simulink model "version 1.0"  (R2020a)
settings: Solver=FixedStepAuto  StartTime=0.0  StopTime=10.0  FixedStep=1e-3  RelTol=1e-3  EnableMultiTasking=on
settings Model: ExtModeTrigDuration=5  Creator=qasim  LastModifiedBy=qasim
settings OptimizationCC: EnhancedBackFolding=on  PassReuseOutputArgsAs=Individual arguments  ZeroExternalMemoryAtStartup=off  ZeroInternalMemoryAtStartup=off  MaxStackSize=64  OptimizeBlockOrder=speed  DifferentSizesBufferReuse=on  OptimizationCustomize=off  EfficientTunableParamExpr=on
settings DebuggingCC: ParameterTunabilityLossMsg=error
settings HardwareCC: ProdBitPerPointer=32  ProdBitPerSizeT=32  ProdBitPerPtrDiffT=32  ProdLargestAtomicInteger=Long  ProdLargestAtomicFloat=Double  ProdWordSize=32  ProdHWDeviceType=ARM Compatible->ARM Cortex
settings SFSimCC: MATLABDynamicMemAlloc=off
settings RTWCC: SystemTargetFile=ert.tlc  HardwareBoard=NXP FRDM-K64F  TemplateMakefile=ert_default_tmf  Toolchain=GNU Tools for ARM Embedded Processors
settings CodeAppCC: ForceParamTrailComments=on  IgnoreCustomStorageClasses=off  OperatorAnnotations=on  SimulinkDataObjDesc=on  SFDataObjDesc=on  InsertBlockDesc=on

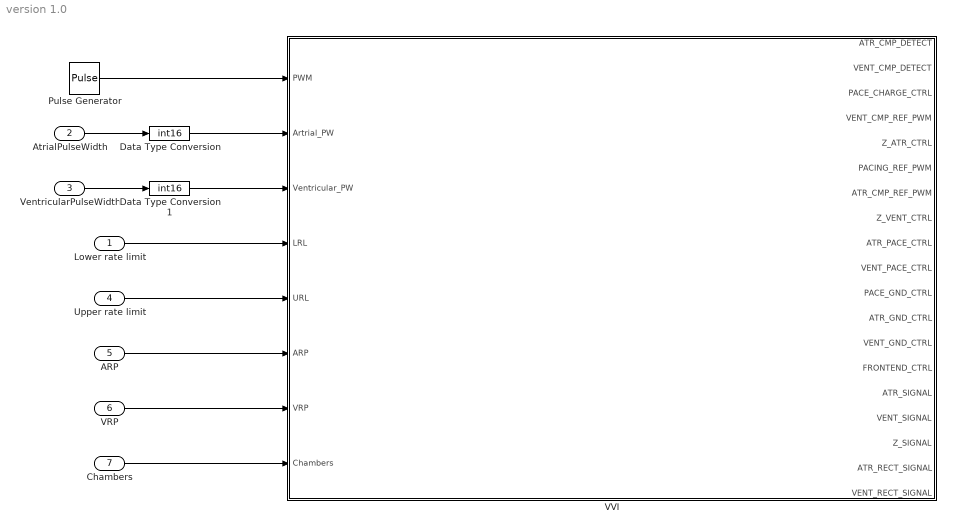
== system version 1.0 ==
  Lower rate limit : Inport
  AtrialPulseWidth : Inport  Port=2
  VentricularPulseWidth : Inport  Port=3
  Upper rate limit : Inport  Port=4
  ARP : Inport  Port=5
  VRP : Inport  Port=6
  Chambers : Inport  Port=7
  Data Type Conversion : DataTypeConversion  OutDataTypeStr=int16
  Data Type Conversion1 : DataTypeConversion  OutDataTypeStr=int16
  Pulse Generator : DiscretePulseGenerator  PulseType=Time based  Period=10  PulseWidth=5
  VVI : Stateflow chart  TreatAsAtomicUnit=on
  wires:
  Pulse Generator/1 -> VVI/1(PWM)
  Lower rate limit/1 -> VVI/4(LRL)
  AtrialPulseWidth/1 -> Data Type Conversion/1
  Data Type Conversion/1 -> VVI/2(Artrial_PW)
  Data Type Conversion1/1 -> VVI/3(Ventricular_PW)
  VentricularPulseWidth/1 -> Data Type Conversion1/1
  Upper rate limit/1 -> VVI/5(URL)
  Chambers/1 -> VVI/8(Chambers)
  VRP/1 -> VVI/7(VRP)
  ARP/1 -> VVI/6(ARP)

== stateflow chart version 1.0/VVI ==
  state INIT
    entry:
    ATR_CMP_DETECT;
    VENT_CMP_DETECT;
    PACE_CHARGE_CTRL = false;
    VENT_CMP_REF_PWM = 90;
    Z_ATR_CTRL = false;
    PACING_REF_PWM;
    ATR_CMP_REF_PWM = 90;
    Z_VENT_CTRL = false;
    ATR_PACE_CTRL = false;
    VENT_PACE_CTRL = false;
    PACE_GND_CTRL = false;
    ATR_GND_CTRL = false;
    VENT_GND_CTRL = false;
    FRONTEND_CTRL = true;
    ATR_SIGNAL = false;
    VENT_SIGNAL = false;
    Z_SIGNAL = false;
    ATR_RECT_SIGNAL = false;
    VENT_RECT_SIGNAL = false;
  state ?
  state ?
  state ?
  state ?
  (default) -> INIT
  INIT -> ? : [Chambers ==1 | Chambers = 0]
  data: PWM input; Artrial_PW input; Ventricular_PW input; LRL input; URL input; ARP input; VRP input; Chambers input; ATR_CMP_DETECT output; VENT_CMP_DETECT output; PACE_CHARGE_CTRL output; VENT_CMP_REF_PWM output; Z_ATR_CTRL output; PACING_REF_PWM output; ATR_CMP_REF_PWM output; Z_VENT_CTRL output; ATR_PACE_CTRL output; VENT_PACE_CTRL output; PACE_GND_CTRL output; ATR_GND_CTRL output; VENT_GND_CTRL output; FRONTEND_CTRL output; ATR_SIGNAL output; VENT_SIGNAL output; Z_SIGNAL output; ATR_RECT_SIGNAL output; VENT_RECT_SIGNAL output
